simulink model "gravityComp"  (R2023b)
settings: Solver=FixedStepAuto  StartTime=0.0  StopTime=15  FixedStep=sampleTime  MaxStep=0.01  RelTol=1e-3
values from neighbouring files (symbols this model uses):
  distortionMatrix = eye(nJoints,nJoints) + noiseMagnitude * randomMatrix    [gravComp_main.m]
  Kp = 5 * eye(nJoints,nJoints)    [gravComp_main.m]
  myRob = loadrobot("universalUR5")    [gravComp_main.m]
  q0 = [2.6016    3.9410   -1.1573   -2.3712   -1.9481    2.0898]'    [gravComp_main.m]
  q0dot = zeros(nJoints,1)    [gravComp_main.m]
  qF = [4.5374    3.2896    2.3615    4.6651   -4.1118    4.4010]'    [gravComp_main.m]
libraries: robotmaniplib x4
settings Model: SimulationMode=accelerator  Creator=ggi01  LastModifiedBy=ggi01
settings SolverCC: AlgebraicLoopSolver=TrustRegion
settings DebuggingCC: UnconnectedInputMsg=warning  UnconnectedOutputMsg=warning  UnconnectedLineMsg=warning
settings ModelReferenceCC: EnableRefExpFcnMdlSchedulingChecks=on
settings RTWCC: DLArmComputeVersion=19.05

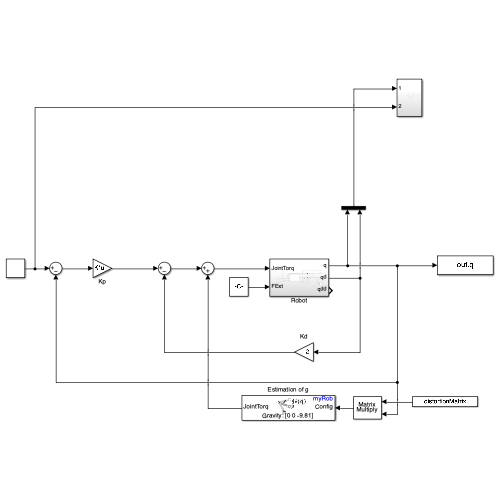
[thumbnail: Simulink's stored preview of the top-level diagram]
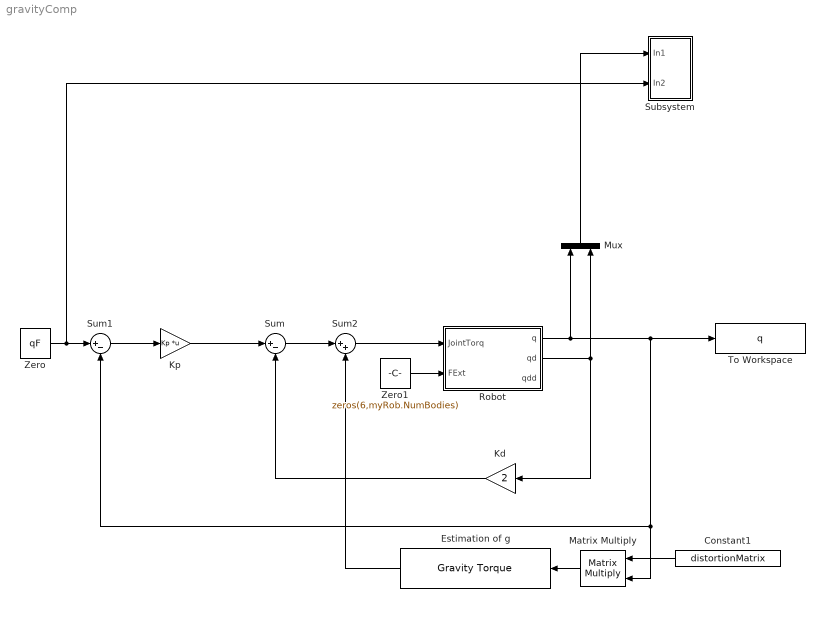
== system gravityComp ==
  Constant1 : Constant  Value=distortionMatrix
  Estimation of g : robotmaniplib/Gravity Torque  RigidBodyTree=myRob  SimulateUsing=Code generation
  Kd : Gain  Gain=2
  Kp : Gain  Gain=Kp  Multiplication=Matrix(K*u)
  Matrix Multiply : Product  Multiplication=Matrix(*)
  Mux : Mux  Inputs=2
  Robot : Subsystem
  Subsystem : Subsystem
  Sum : Sum  Inputs=|+-
  Sum1 : Sum  Inputs=|+-
  Sum2 : Sum  Inputs=|++
  To Workspace : ToWorkspace  VariableName=q  SampleTime=-1
  Zero : Constant  Value=qF  VectorParams1D=off  OutDataTypeStr=Inherit: Inherit via back propagation
  Zero1 : Constant  Value=zeros(6,myRob.NumBodies)  VectorParams1D=off  OutDataTypeStr=Inherit: Inherit via back propagation
  wires:
  Zero1/1 -> Robot/2(FExt)
  Robot/1(q) -> Matrix Multiply/2, Sum1/2, To Workspace/1, Mux/1
  Kd/1 -> Sum/2
  Kp/1 -> Sum/1
  Sum1/1 -> Kp/1
  Robot/2(qd) -> Kd/1, Mux/2
  Zero/1 -> Subsystem/2(In2), Sum1/1
  Sum/1 -> Sum2/1
  Sum2/1 -> Robot/1(JointTorq)
  Estimation of g/1 -> Sum2/2
  Constant1/1 -> Matrix Multiply/1
  Matrix Multiply/1 -> Estimation of g/1
  Mux/1 -> Subsystem/1(In1)

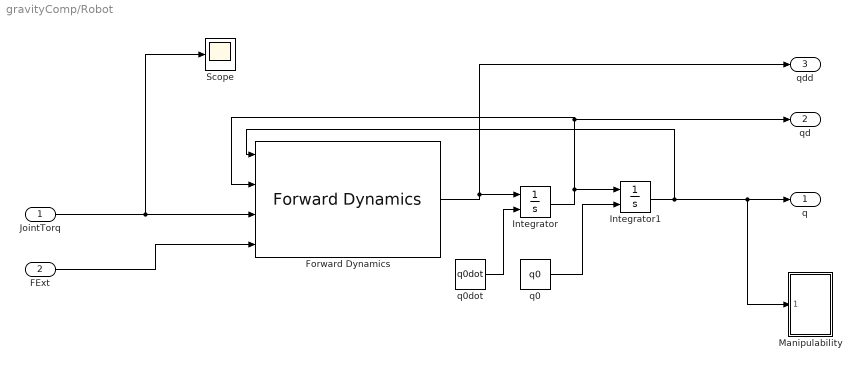
== system gravityComp/Robot ==
  JointTorq : Inport
  FExt : Inport  Port=2
  Forward Dynamics : robotmaniplib/Forward Dynamics  RigidBodyTree=myRob  SimulateUsing=Code generation
  Integrator : Integrator  InitialConditionSource=external
  Integrator1 : Integrator  InitialConditionSource=external
  Manipulability : Subsystem
  Scope : Scope
  q0 : Constant  Value=q0
  q0dot : Constant  Value=q0dot
  q : Outport
  qd : Outport  Port=2
  qdd : Outport  Port=3
  wires:
  q0/1 -> Integrator1/2
  Forward Dynamics/1 -> qdd/1, Integrator/1
  FExt/1 -> Forward Dynamics/4
  JointTorq/1 -> Scope/1, Forward Dynamics/3
  Integrator/1 -> qd/1, Forward Dynamics/2, Integrator1/1
  Integrator1/1 -> Manipulability/1(Config), q/1, Forward Dynamics/1
  q0dot/1 -> Integrator/2

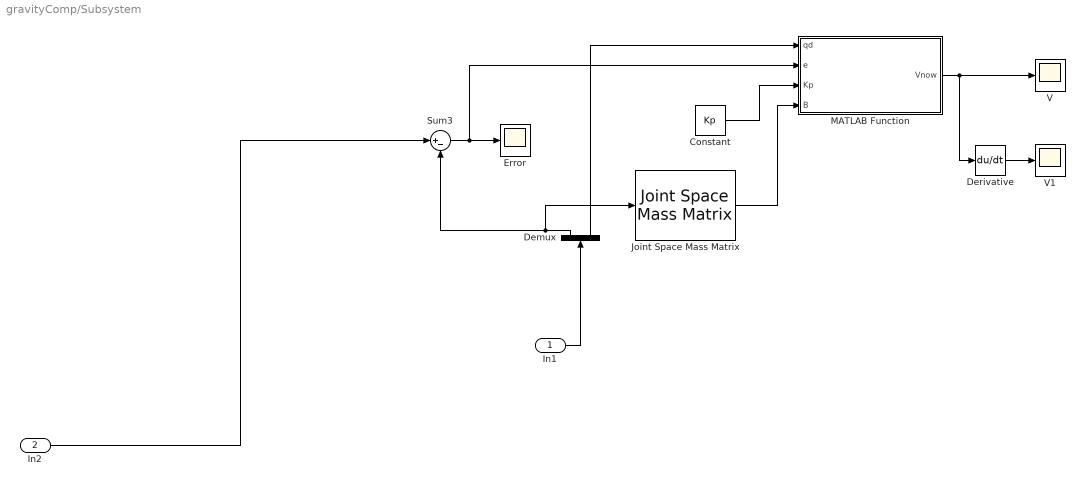
== system gravityComp/Subsystem ==
  In1 : Inport
  In2 : Inport  Port=2
  Constant : Constant  Value=Kp
  Demux : Demux  Outputs=2
  Derivative : Derivative
  Error : Scope
  Joint Space Mass Matrix : robotmaniplib/Joint Space Mass Matrix  RigidBodyTree=myRob  SimulateUsing=Code generation
  MATLAB Function : MATLAB Function  TreatAsAtomicUnit=on
  Sum3 : Sum  Inputs=|+-
  V : Scope
  V1 : Scope
  wires:
  In2/1 -> Sum3/1
  In1/1 -> Demux/1
  Derivative/1 -> V1/1
  MATLAB Function/1(Vnow) -> Derivative/1, V/1
  Sum3/1 -> MATLAB Function/2(e), Error/1
  Constant/1 -> MATLAB Function/3(Kp)
  Joint Space Mass Matrix/1 -> MATLAB Function/4(B)
  Demux/1 -> Joint Space Mass Matrix/1, Sum3/2
  Demux/2 -> MATLAB Function/1(qd)

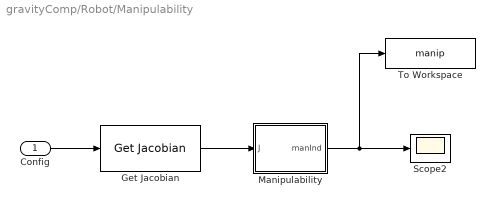
== system gravityComp/Robot/Manipulability ==
  Config : Inport
  Get Jacobian : robotmaniplib/Get Jacobian  RigidBodyTree=myRob  EndEffector=tool0  SimulateUsing=Interpreted execution
  Manipulability : MATLAB Function  TreatAsAtomicUnit=on
  Scope2 : Scope
  To Workspace : ToWorkspace  VariableName=manip  SaveFormat=Timeseries  SampleTime=-1
  wires:
  Config/1 -> Get Jacobian/1
  Manipulability/1(manInd) -> To Workspace/1, Scope2/1
  Get Jacobian/1 -> Manipulability/1(J)

== matlab function gravityComp/Robot/Manipulability/Manipulability ==
  data: J input; manInd output
function manInd = fcn(J)
    manInd = sqrt(det(J * J'));

== matlab function gravityComp/Subsystem/MATLAB Function ==
  data: qd input; Vnow output; e input; Kp input; B input
function Vnow = lyapunovCandidateWrap(qd,e,Kp,B)
Vnow = lyapunovCandidate(qd,e,Kp,B);
